simulink model "nonlinear_simulation_minitvc_v4"  (R2024b)
settings: Solver=ode15s  StartTime=0.0  StopTime=30.0  MinStep=0.001  RelTol=1e-3
values from neighbouring files (symbols this model uses):
  a = 0.1    [linear_controller_compute_no_integ.m]
  g = 9.807    [linear_controller_compute_no_integ.m]    (also in new_strategy.m = 9.81)
  J_mat = [Jx, 0, 0 ... (first row only)    [linear_controller_compute_no_integ.m]
  J_mat_inv = J_mat ^ -1    [linear_controller_compute_no_integ.m]
  K_hov0 = lqr(sys_red, Q_red, R)    [linear_controller_compute_no_integ.m]
  K_pos = lqr(sys_hor, Q_pos, R_pos)    [linear_controller_compute_no_integ.m]
  Km = 0.00016    [linear_controller_compute_no_integ.m]
  Kt = 0.001    [linear_controller_compute_no_integ.m]
  m = 0.75    [linear_controller_compute_no_integ.m]    (also in new_strategy.m = 1)
libraries: matrix_library x1
settings Model: Creator=yoonj  LastModifiedBy=yh583
settings SolverCC: MaxConsecutiveMinStep=2

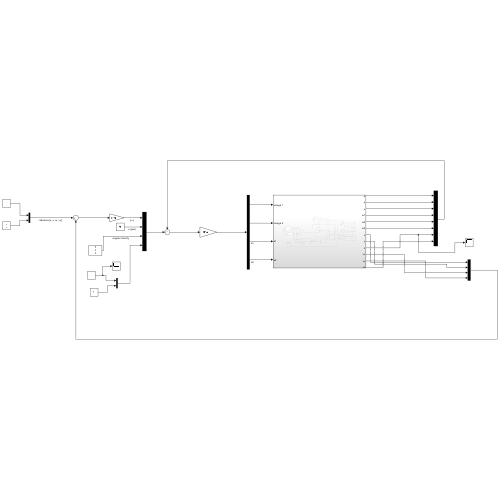
[thumbnail: Simulink's stored preview of the top-level diagram]
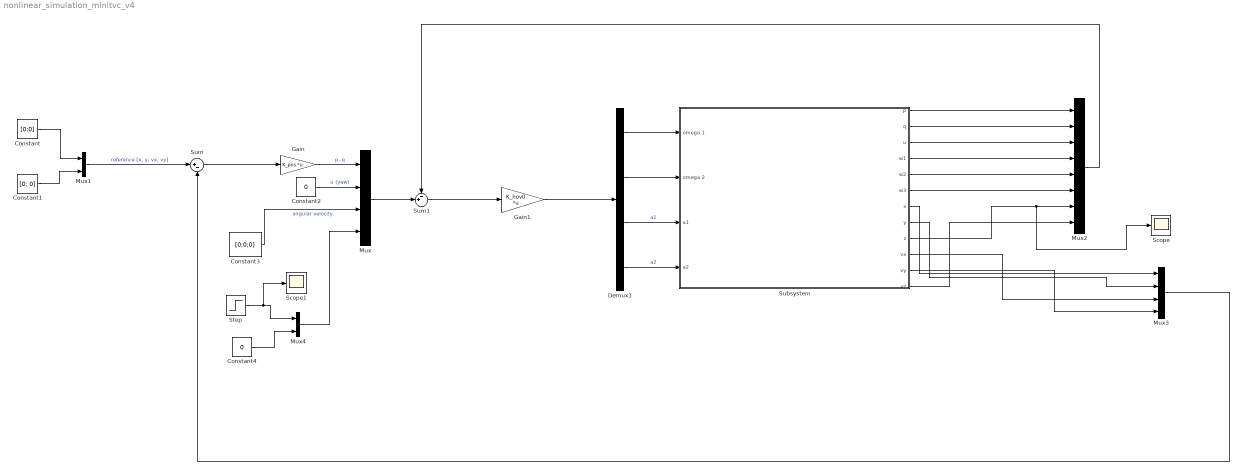
== system nonlinear_simulation_minitvc_v4 ==
  Constant : Constant  Value=[0;0]  VectorParams1D=off
  Constant1 : Constant  Value=[0; 0]  VectorParams1D=off
  Constant2 : Constant  Value=0
  Constant3 : Constant  Value=[0;0;0]  VectorParams1D=off
  Constant4 : Constant  Value=0
  Demux1 : Demux
  Gain : Gain  Gain=K_pos  Multiplication=Matrix(K*u)
  Gain1 : Gain  Gain=K_hov0  Multiplication=Matrix(K*u)
  Mux : Mux
  Mux1 : Mux  Inputs=2
  Mux2 : Mux  Inputs=8
  Mux3 : Mux
  Mux4 : Mux  Inputs=2
  Scope : Scope
  Scope1 : Scope
  Step : Step  SampleTime=0
  Subsystem : Subsystem
  Sum : Sum  Inputs=|+-
  Sum1 : Sum  Inputs=-+|
  wires:
  Gain/1 -> Mux/1  "p, q"
  Constant/1 -> Mux1/1
  Constant1/1 -> Mux1/2
  Mux1/1 -> Sum/1  "reference [x, y, vx, vy]"
  Constant2/1 -> Mux/2  "u (yaw)"
  Constant3/1 -> Mux/3  "angular velocity"
  Gain1/1 -> Demux1/1
  Mux/1 -> Sum1/2
  Demux1/1 -> Subsystem/1(omega 1)
  Demux1/2 -> Subsystem/2(omega 2)
  Demux1/3 -> Subsystem/3(a1)  "a1"
  Demux1/4 -> Subsystem/4(a2)  "a2"
  Subsystem/1(p) -> Mux2/1
  Subsystem/2(q) -> Mux2/2
  Subsystem/3(u) -> Mux2/3
  Subsystem/4(w1) -> Mux2/4
  Subsystem/5(w2) -> Mux2/5
  Subsystem/6(w3) -> Mux2/6
  Subsystem/9(z) -> Scope/1, Mux2/7
  Subsystem/12(vz) -> Mux2/8
  Subsystem/7(x) -> Mux3/1
  Subsystem/8(y) -> Mux3/2
  Subsystem/10(vx) -> Mux3/3
  Subsystem/11(vy) -> Mux3/4
  Mux2/1 -> Sum1/1
  Mux3/1 -> Sum/2
  Step/1 -> Scope1/1, Mux4/1
  Constant4/1 -> Mux4/2
  Mux4/1 -> Mux/4
  Sum1/1 -> Gain1/1
  Sum/1 -> Gain/1

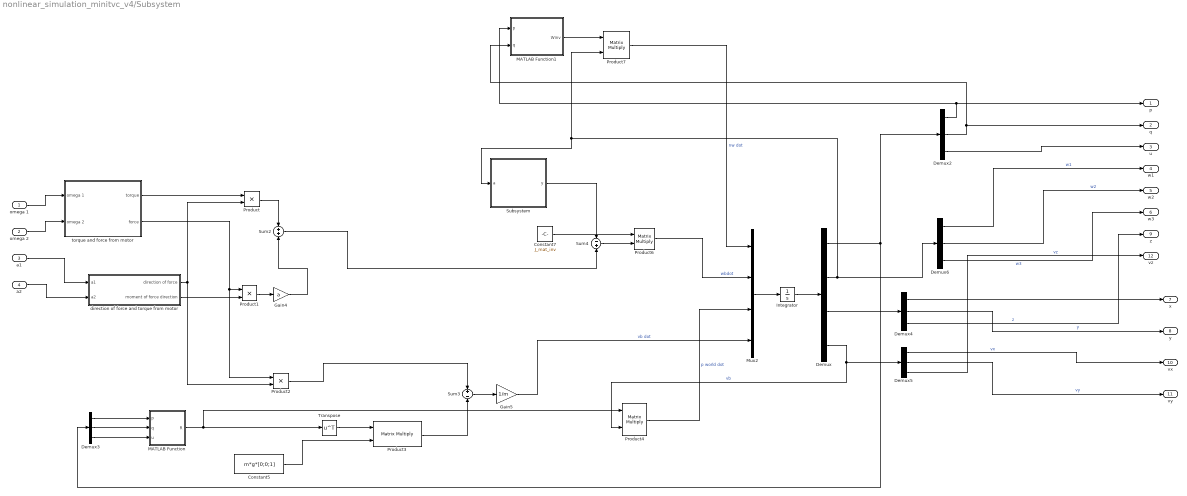
== system nonlinear_simulation_minitvc_v4/Subsystem ==
  omega 1 : Inport
  omega 2 : Inport  Port=2
  a1 : Inport  Port=3
  a2 : Inport  Port=4
  Constant5 : Constant  Value=m*g*[0;0;1]  VectorParams1D=off
  Constant7 : Constant  Value=J_mat_inv  VectorParams1D=off
  Demux : Demux
  Demux{2..6} (5 alike) : Demux  Outputs=3
  Gain4 : Gain  Gain=a
  Gain5 : Gain  Gain=1/m
  Integrator : Integrator  InitialCondition=[0; 0; 0; 0; 0; 0; 0; 0; 0; 0; 0; 0]
  MATLAB Function : MATLAB Function  TreatAsAtomicUnit=on
  MATLAB Function1 : MATLAB Function  TreatAsAtomicUnit=on
  Mux2 : Mux
  Product : Product
  Product1 : Product
  Product2 : Product
  Product{3..4,6..7} (4 alike) : Product  Multiplication=Matrix(*)
  Subsystem : Subsystem
  Sum2 : Sum  Inputs=+|+
  Sum3 : Sum  Inputs=+|-
  Sum4 : Sum  Inputs=-|+
  Transpose : Math  Operator=transpose
  direction of force and torque from motor : Subsystem
  torque and force from motor : Subsystem
  p : Outport
  q : Outport  Port=2
  u : Outport  Port=3
  w1 : Outport  Port=4
  w2 : Outport  Port=5
  w3 : Outport  Port=6
  x : Outport  Port=7
  y : Outport  Port=8
  z : Outport  Port=9
  vx : Outport  Port=10
  vy : Outport  Port=11
  vz : Outport  Port=12
  wires:
  Demux3/3 -> MATLAB Function/3(u)
  Gain5/1 -> Mux2/4  "vb dot"
  Demux2/3 -> u/1
  Gain4/1 -> Sum2/2
  a1/1 -> direction of force and torque from motor/1(a1)
  MATLAB Function1/1(Winv) -> Product7/1
  Sum3/1 -> Gain5/1
  MATLAB Function/1(R) -> Product4/1, Transpose/1
  direction of force and torque from motor/2(moment of force direction) -> Product1/2
  Product7/1 -> Mux2/1  "nw dot"
  Product4/1 -> Mux2/3  "p world dot"
  Demux/2 -> Product7/2, Subsystem/1(a), Demux6/1
  Product3/1 -> Sum3/2
  Demux2/1 -> p/1, MATLAB Function1/1(p)
  Demux4/3 -> z/1  "z"
  direction of force and torque from motor/1(direction of force) -> Product/2, Product2/2
  torque and force from motor/2(force) -> Product1/1, Product2/1
  Transpose/1 -> Product3/1
  Product/1 -> Sum2/1
  Constant5/1 -> Product3/2
  Demux6/1 -> w1/1  "w1"
  a2/1 -> direction of force and torque from motor/2(a2)
  Product2/1 -> Sum3/1
  Demux4/1 -> x/1
  Integrator/1 -> Demux/1
  Product1/1 -> Gain4/1
  torque and force from motor/1(torque) -> Product/1
  omega 2/1 -> torque and force from motor/2(omega 2)
  Product6/1 -> Mux2/2  "wbdot"
  Sum2/1 -> Sum4/2
  Demux/4 -> Product4/2, Demux5/1  "vb"
  Demux3/1 -> MATLAB Function/1(p)
  Constant7/1 -> Product6/1
  Demux3/2 -> MATLAB Function/2(q)
  omega 1/1 -> torque and force from motor/1(omega 1)
  Sum4/1 -> Product6/2
  Mux2/1 -> Integrator/1
  Demux2/2 -> q/1, MATLAB Function1/2(q)
  Demux/3 -> Demux4/1
  Demux6/2 -> w2/1  "w2"
  Demux/1 -> Demux3/1, Demux2/1
  Demux5/3 -> vz/1  "vz"
  Demux5/1 -> vx/1  "vx"
  Demux5/2 -> vy/1  "vy"
  Demux6/3 -> w3/1  "w3"
  Demux4/2 -> y/1  "y"
  Subsystem/1(y) -> Sum4/1

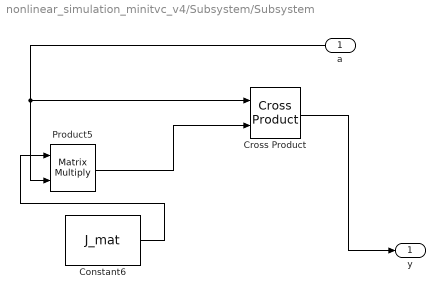
== system nonlinear_simulation_minitvc_v4/Subsystem/Subsystem ==
  a : Inport
  Constant6 : Constant  Value=J_mat  VectorParams1D=off
  Cross Product : matrix_library/Cross Product
  Product5 : Product  Multiplication=Matrix(*)
  y : Outport
  wires:
  Constant6/1 -> Product5/1
  Product5/1 -> Cross Product/2
  Cross Product/1 -> y/1
  a/1 -> Cross Product/1, Product5/2

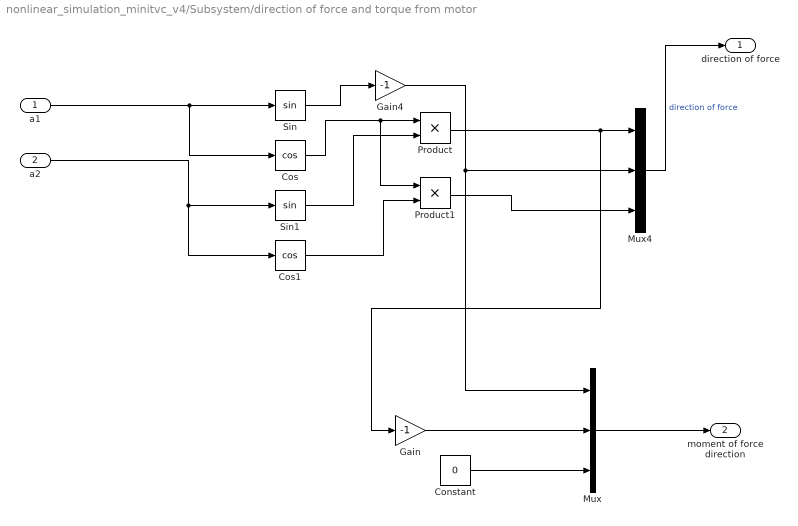
== system nonlinear_simulation_minitvc_v4/Subsystem/direction of force and torque from motor ==
  a1 : Inport
  a2 : Inport  Port=2
  Constant : Constant  Value=0
  Cos : Trigonometry  Operator=cos
  Cos1 : Trigonometry  Operator=cos
  Gain : Gain  Gain=-1
  Gain4 : Gain  Gain=-1
  Mux : Mux  Inputs=3
  Mux4 : Mux  Inputs=3
  Product : Product
  Product1 : Product
  Sin : Trigonometry
  Sin1 : Trigonometry
  direction of force : Outport
  moment of force direction : Outport  Port=2
  wires:
  Sin1/1 -> Product/2
  Product/1 -> Gain/1, Mux4/1
  Gain4/1 -> Mux/1, Mux4/2
  a1/1 -> Cos/1, Sin/1
  a2/1 -> Cos1/1, Sin1/1
  Sin/1 -> Gain4/1
  Cos/1 -> Product1/1, Product/1
  Cos1/1 -> Product1/2
  Product1/1 -> Mux4/3
  Mux4/1 -> direction of force/1  "direction of force"
  Gain/1 -> Mux/2
  Constant/1 -> Mux/3
  Mux/1 -> moment of force direction/1

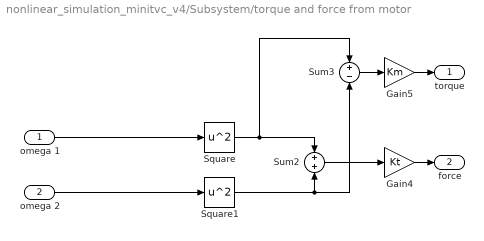
== system nonlinear_simulation_minitvc_v4/Subsystem/torque and force from motor ==
  omega 1 : Inport
  omega 2 : Inport  Port=2
  Gain4 : Gain  Gain=Kt
  Gain5 : Gain  Gain=Km
  Square : Math  Operator=square
  Square1 : Math  Operator=square
  Sum2 : Sum  Inputs=+|+
  Sum3 : Sum  Inputs=+|-
  torque : Outport
  force : Outport  Port=2
  wires:
  Square1/1 -> Sum3/2, Sum2/2
  omega 2/1 -> Square1/1
  Sum3/1 -> Gain5/1
  Square/1 -> Sum3/1, Sum2/1
  Gain5/1 -> torque/1
  Sum2/1 -> Gain4/1
  Gain4/1 -> force/1
  omega 1/1 -> Square/1

== matlab function nonlinear_simulation_minitvc_v4/Subsystem/MATLAB Function ==
  data: p input; q input; u input; R output
function R = rotation(p,q,u)
    R = [cos(q)*cos(u), sin(p)*sin(q)*cos(u)-cos(p)*sin(u), cos(p)*sin(q)*cos(u)+sin(p)*sin(u) ;
         cos(q)*sin(u), sin(p)*sin(q)*sin(u)+cos(p)*cos(u), cos(p)*sin(q)*sin(u)-sin(p)*cos(u) ;
         -sin(q),       sin(p)*cos(q),                      cos(p)*cos(q)                     ];

== matlab function nonlinear_simulation_minitvc_v4/Subsystem/MATLAB Function1 ==
  data: p input; q input; Winv output
function Winv = angv_to_orientation(p,q)
Winv = [1, (sin(p)*sin(q))/cos(q), (cos(p)*sin(q))/cos(q);
        0,                 cos(p),                -sin(p);
        0,          sin(p)/cos(q),          cos(p)/cos(q)];
